simulink model "planning"  (R2020a)
settings: Solver=VariableStepAuto  StartTime=0.0  StopTime=inf  RelTol=1e-3
values from neighbouring files (symbols this model uses):
  K = 0.5    [main5_simulink.m]    (also in main5_simulink_exp.m)
  KD = 3    [main5_simulink.m]    (also in main5_simulink_exp.m)
  KP = 1.2    [main5_simulink.m]    (also in main5_simulink_exp.m)
  Ld = 20    [main5_simulink.m]    (also in main5_simulink_exp.m = 10)
  psi_0 = 0    [main5_simulink.m]    (also in main5_simulink_exp.m)
  T = minspantree(Gr)    [MST_plan.m]    (also in MST_plan_hex.m; MST_plan_hex_out.m; MST_plan_out.m; OCP_plan.m = opti.variable(1,1))
  V = 2.5    [main5_simulink.m]    (also in main5_simulink_exp.m)
  waypoints = [waypoints;[pos1sol_prov(end) pos2sol_prov(end)]]    [Boustro_backtrack_plan.m]    (also in OCP_plan.m; OCP_plan4.m; main5_simulink.m = scale*[pos1sol_ocp pos2sol_ocp]; main5_simulink_exp.m = scale*[pos1sol_mst, pos2sol_mst])
  x0 = waypoints(1,1)    [main5_simulink.m]    (also in main5_simulink_exp.m)
  y0 = waypoints(1,2)    [main5_simulink.m]    (also in main5_simulink_exp.m)
settings Model: Creator=User  LastModifiedBy=User

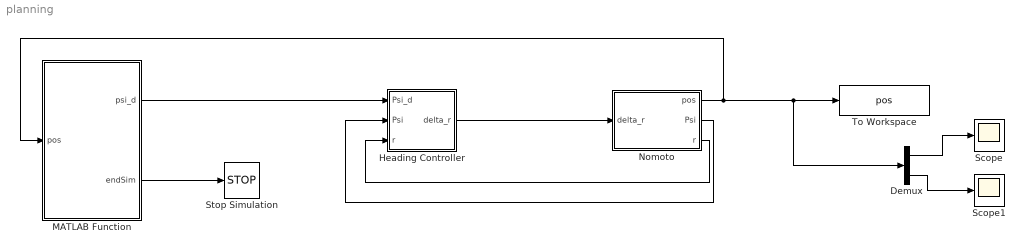
== system planning ==
  Demux : Demux  Outputs=2
  Heading Controller : Subsystem
  MATLAB Function : MATLAB Function  TreatAsAtomicUnit=on
  Nomoto : Subsystem
  Scope : Scope
  Scope1 : Scope
  Stop Simulation : Stop
  To Workspace : ToWorkspace  VariableName=pos  SampleTime=-1
  wires:
  Nomoto/1(pos) -> Demux/1, To Workspace/1, MATLAB Function/1(pos)
  MATLAB Function/1(psi_d) -> Heading Controller/1(Psi_d)
  Nomoto/2(Psi) -> Heading Controller/2(Psi)
  Nomoto/3(r) -> Heading Controller/3(r)
  Heading Controller/1(delta_r) -> Nomoto/1(delta_r)
  MATLAB Function/2(endSim) -> Stop Simulation/1
  Demux/1 -> Scope/1
  Demux/2 -> Scope1/1

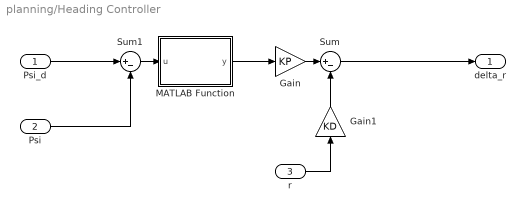
== system planning/Heading Controller ==
  Psi_d : Inport
  Psi : Inport  Port=2
  r : Inport  Port=3
  Gain : Gain  Gain=KP
  Gain1 : Gain  Gain=KD
  MATLAB Function : MATLAB Function  TreatAsAtomicUnit=on
  Sum : Sum  Inputs=|+-
  Sum1 : Sum  Inputs=|+-
  delta_r : Outport
  wires:
  Gain/1 -> Sum/1
  r/1 -> Gain1/1
  Psi/1 -> Sum1/2
  Gain1/1 -> Sum/2
  Sum/1 -> delta_r/1
  Psi_d/1 -> Sum1/1
  Sum1/1 -> MATLAB Function/1(u)
  MATLAB Function/1(y) -> Gain/1

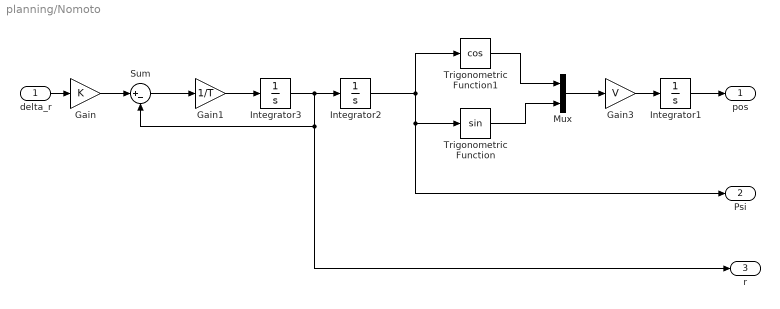
== system planning/Nomoto ==
  delta_r : Inport
  Gain : Gain  Gain=K
  Gain1 : Gain  Gain=1/T
  Gain3 : Gain  Gain=V
  Integrator1 : Integrator  InitialCondition=[x0;y0]
  Integrator2 : Integrator  InitialCondition=psi_0
  Integrator3 : Integrator
  Mux : Mux  Inputs=2
  Sum : Sum  Inputs=|+-
  Trigonometric Function : Trigonometry
  Trigonometric Function1 : Trigonometry  Operator=cos
  pos : Outport
  Psi : Outport  Port=2
  r : Outport  Port=3
  wires:
  Gain/1 -> Sum/1
  Gain3/1 -> Integrator1/1
  Integrator3/1 -> r/1, Sum/2, Integrator2/1
  Sum/1 -> Gain1/1
  delta_r/1 -> Gain/1
  Gain1/1 -> Integrator3/1
  Mux/1 -> Gain3/1
  Trigonometric Function1/1 -> Mux/1
  Integrator2/1 -> Trigonometric Function/1, Psi/1, Trigonometric Function1/1
  Trigonometric Function/1 -> Mux/2
  Integrator1/1 -> pos/1

== matlab function planning/Heading Controller/MATLAB Function ==
  data: u input; y output
function y = fcn(u)

y = mod(u+pi,2*pi)-pi;

== matlab function planning/MATLAB Function ==
  settings: updateMethod=DISCRETE
  data: pos input; psi_d output; waypoints parameter; Ld parameter; endSim output
function [psi_d,endSim] = purePursuit(pos, waypoints, Ld)
% pos = [x y]  (se precisar de psi acrescente depois)
persistent idx
if isempty(idx); idx = 1; end

N = size(waypoints,1);

%% --- 1. Avançar idx se já cruzámos o plano perpendicular a p1 ---
while idx < N
    p0  = waypoints(idx   ,:);
    p1  = waypoints(idx+1 ,:);
    seg = p1 - p0;

    % produto interno: >0  ⇒ pos está “depois” de p1 ao longo do seg
    if dot(pos' - p1 , seg) >  0.0 || norm(waypoints(idx+1,:) - pos') < Ld          % passou
        idx = idx + 1;
    else
        break                               % ainda não passou
    end
end

%% --- 2. Definir alvo de look-ahead ao longo do mesmo segmento ---
if idx >= N          % último ponto atingido
    p1  = waypoints(idx ,:);
    
    psi_d  = atan2( (p1(2)-pos(2)), (p1(1)-pos(1)) );
    endSim = 1;
    return
end

p0  = waypoints(idx   ,:);
p1  = waypoints(idx+1 ,:);
seg = p1 - p0;
Lseg = norm(seg);

% Projecção ortogonal
s    = dot(pos' - p0, seg) / Lseg;      % distância ao longo da recta
s    = max(0, min(Lseg, s));            % clamp 0…Lseg
proj = p0 + (s / Lseg) * seg;

% Ponto carrot
look = proj + (Ld * seg / Lseg);        % desloca Ld à frente
dir  = look - pos';

%% --- 3. Ângulo desejado ---
psi_d  = atan2(dir(2), dir(1));
endSim = 0;
end
